simulink model "DCmotor_LeadLag"  (R2025b)
settings: Solver=VariableStepAuto  StartTime=0.0  StopTime=20  RelTol=1e-3
undefined symbols (not defined in the file): K, k1, k2, K_c, tau
settings Model: Creator=User  LastModifiedBy=User

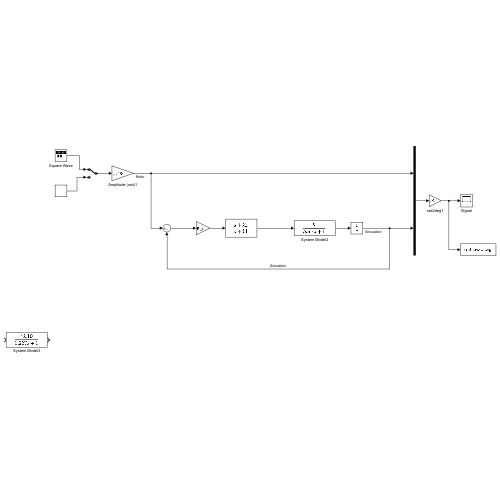
[thumbnail: Simulink's stored preview of the top-level diagram]
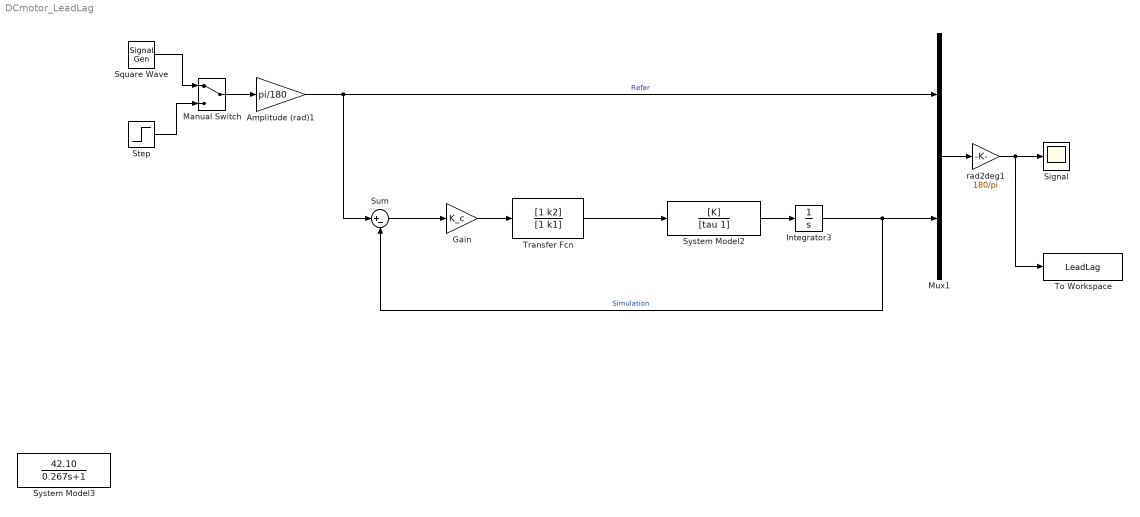
== system DCmotor_LeadLag ==
  Amplitude (rad)1 : Gain  Gain=pi/180
  Gain : Gain  Gain=K_c
  Integrator3 : Integrator
  Manual Switch : ManualSwitch
  Mux1 : Mux  Inputs=2
  Signal : Scope
      settings: TimeSpan=20  ActiveDisplayYMinimum=-153.10943251525291  ActiveDisplayYMaximum=99.850321227035678  DataLoggingMaxPoints=25000  DataLoggingSaveFormat=Array
  Square Wave : SignalGenerator  WaveForm=square  Amplitude=45  Frequency=0.1
  Step : Step  SampleTime=0
  Sum : Sum  Inputs=|+-
  System Model2 : TransferFcn  Numerator=[K]  Denominator=[tau 1]
  System Model3 : TransferFcn  Numerator=42.10  Denominator=[0.267 1]
  To Workspace : ToWorkspace  VariableName=LeadLag  SaveFormat=Timeseries  SampleTime=-1
  Transfer Fcn : TransferFcn  Numerator=[1 k2]  Denominator=[1 k1]
  rad2deg1 : Gain  Gain=180/pi
  wires:
  Integrator3/1 -> Sum/2, Mux1/2  "Simulation"
  Mux1/1 -> rad2deg1/1
  Step/1 -> Manual Switch/2
  Amplitude (rad)1/1 -> Sum/1, Mux1/1  "Refer"
  rad2deg1/1 -> To Workspace/1, Signal/1
  Manual Switch/1 -> Amplitude (rad)1/1
  System Model2/1 -> Integrator3/1
  Square Wave/1 -> Manual Switch/1
  Gain/1 -> Transfer Fcn/1
  Sum/1 -> Gain/1
  Transfer Fcn/1 -> System Model2/1
